simulink model "DTNS"  (R2022a)
settings: Solver=FixedStepDiscrete  StartTime=0.0  StopTime=0.4  FixedStep=0.04  RelTol=1e-3
PreLoadFcn:
  | listing = dir;
  | if (contains([listing.name], 'MAP')) &&  (contains([listing.name], 'DTNS.slx'))
  |     addpath('./AGR', './TRN', './TCAF', './MAP');
  |     addpath('./MAP/MAP_DB');
  | else
  |     warning('[DTNS.slx]는 DTNS 프로젝트 최상단 경로에 위치해야 합니다.');
  | end
  | 
  | load('BusStructureTRN.mat');
  | load('BusStructureLOSR.mat');
  | load('BusStructureHR.mat');
  | load('BusStructureCR.mat');
InitFcn:
  | listing = dir;
  | if (contains([listing.name], 'MAP')) &&  (contains([listing.name], 'DTNS.slx'))
  |     addpath('./AGR', './TRN', './TCAF', './MAP');
  |     addpath('./MAP/MAP_DB');
  | else
  |     warning('[DTNS.slx]는 DTNS 프로젝트 최상단 경로에 위치해야 합니다.');
  | end
  | 
  | load('BusStructureTRN.mat');
  | load('BusStructureLOSR.mat');
  | load('BusStructureHR.mat');
  | load('BusStructureCR.mat');
settings Model: Creator=ASCL  LastModifiedBy=ASCL
settings SolverCC: PositivePriorityOrder=on
settings DataIOCC: SaveOutput=off  SignalLogging=off  DSMLogging=off  SaveTime=off  ReturnWorkspaceOutputs=off
settings OptimizationCC: BlockReduction=off  DefaultParameterBehavior=Inlined  UseDivisionForNetSlopeComputation=on  GainParamInheritBuiltInType=on  UseFloatMulNetSlope=on  ExpressionFolding=off  PassReuseOutputArgsAs=Individual arguments  ZeroExternalMemoryAtStartup=off  ZeroInternalMemoryAtStartup=off  EfficientFloat2IntCast=on  LifeSpan=Inf  OptimizeBlockOrder=speed  DifferentSizesBufferReuse=on  EfficientTunableParamExpr=on
settings DebuggingCC: SignalInfNanChecking=warning  ReadBeforeWriteMsg=EnableAllAsError  WriteAfterWriteMsg=EnableAllAsError  WriteAfterReadMsg=EnableAllAsError  IntegerOverflowMsg=error  ParameterTunabilityLossMsg=error  UniqueDataStoreMsg=error  AssertControl=DisableAll  NonBusSignalsTreatedAsBus=error  SFInvalidInputDataAccessInChartInitDiag=error  SFTransitionOutsideNaturalParentDiag=error  SFUnreachableExecutionPathDiag=error  SFUndirectedBroadcastEventsDiag=error  IntegerSaturationMsg=error
settings HardwareCC: ProdBitPerPointer=32  ProdBitPerSizeT=32  ProdBitPerPtrDiffT=32  ProdLargestAtomicInteger=Long  ProdLargestAtomicFloat=Double  ProdEndianess=BigEndian  ProdWordSize=32  ProdLongLongMode=on  ProdHWDeviceType=Freescale->MPC83xx
settings ModelReferenceCC: ModelReferenceNumInstancesAllowed=Single  PropagateSignalLabelsOutOfModel=off
settings SFSimCC: SimCustomHeaderCode="#include \"MAP.h\""  SimUserSources=MAP.c  SimUserLibraries=WS2_32.LIB  CompileTimeRecursionLimit=0  EnableRuntimeRecursion=off  MATLABDynamicMemAlloc=off
settings RTWCC: SystemTargetFile=ert.tlc  TemplateMakefile=ert_default_tmf  GenerateReport=on  RTWUseSimCustomCode=on  CustomHeaderCode="#include \"MAP.h\""  CustomSource=MAP.c  CustomLibrary=WS2_32.LIB  BuildConfiguration=Faster Runs  IncludeHyperlinkInReport=on  LaunchReport=on  GenerateTraceInfo=on  GenerateTraceReport=on  GenerateTraceReportSl=on  GenerateTraceReportSf=on  GenerateTraceReportEml=on  GenerateCodeMetricsReport=on
settings CodeAppCC: ForceParamTrailComments=on  IgnoreCustomStorageClasses=off  OperatorAnnotations=on  SimulinkDataObjDesc=on  SFDataObjDesc=on  MATLABFcnDesc=on  InsertBlockDesc=on  StateflowObjectComments=on  MATLABSourceComments=on  EnableCustomComments=on  InlinedPrmAccess=Macros  ReqsInCode=on
settings ERTTargetCC: TargetLangStandard=C99 (ISO)  UtilityFuncGeneration=Shared location  GenerateSampleERTMain=on  CombineSignalStateStructs=on  SuppressErrorStatus=on  SupportNonFinite=off  SupportVariableSizeSignals=on  ParenthesesLevel=Standards  CastingMode=Standards  GenerateSharedConstants=off  InlinedParameterPlacement=NonHierarchical  ERTCustomFileTemplate=example_file_process.tlc  RateTransitionBlockCode=Function  PreserveIfCondition=on  ConvertIfToSwitch=off  EnableSignedLeftShifts=off  EnableSignedRightShifts=off

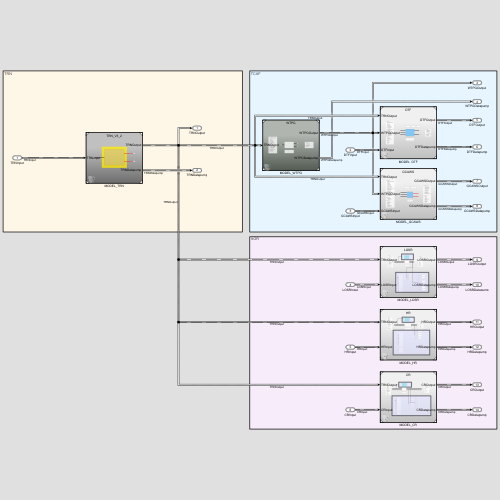
[thumbnail: Simulink's stored preview of the top-level diagram]
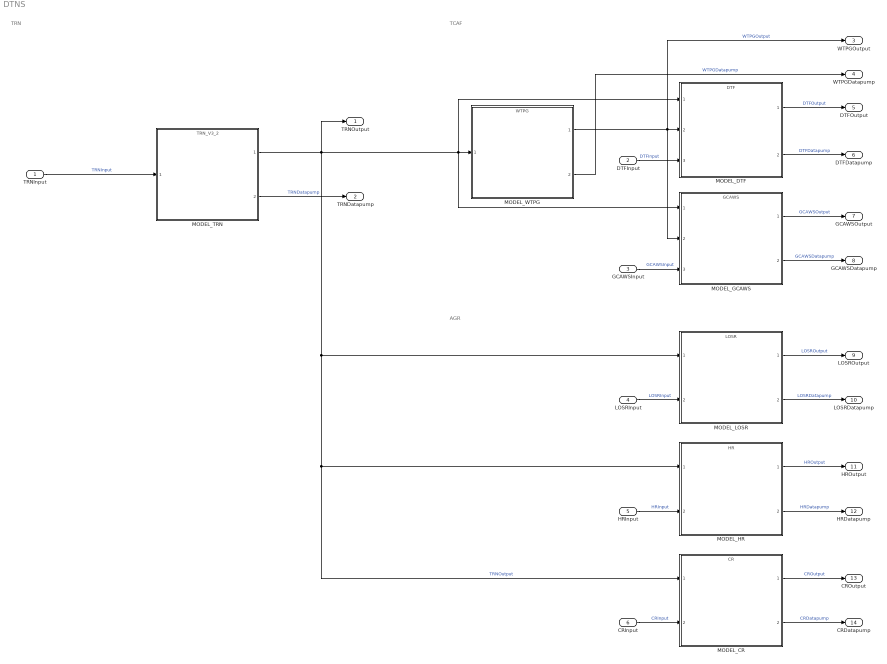
== system DTNS ==
  note: TRN
  note: AGR
  note: TCAF
  TRNInput : Inport  OutDataTypeStr=Bus: TRNInput  SampleTime=0.04  Interpolate=off  BusOutputAsStruct=on
  DTFInput : Inport  Port=2  OutDataTypeStr=Bus: DTFInput  SampleTime=0.04  Interpolate=off  BusOutputAsStruct=on
  GCAWSInput : Inport  Port=3  OutDataTypeStr=Bus: GCAWSInput  SampleTime=0.04  Interpolate=off  BusOutputAsStruct=on
  LOSRInput : Inport  Port=4  OutDataTypeStr=Bus: LOSRInput  SampleTime=0.04  Interpolate=off  BusOutputAsStruct=on
  HRInput : Inport  Port=5  OutDataTypeStr=Bus: HRInput  SampleTime=0.04  Interpolate=off  BusOutputAsStruct=on
  CRInput : Inport  Port=6  OutDataTypeStr=Bus: CRInput  SampleTime=0.04  Interpolate=off  BusOutputAsStruct=on
  MODEL_CR : ModelReference  ModelNameDialog=CR.slx  SimulationMode=Normal  ModelReferenceVersion=1.261
  MODEL_DTF : ModelReference  ModelNameDialog=DTF.slx  SimulationMode=Normal  ModelReferenceVersion=1.441
  MODEL_GCAWS : ModelReference  ModelNameDialog=GCAWS.slx  SimulationMode=Normal  ModelReferenceVersion=1.799
  MODEL_HR : ModelReference  ModelNameDialog=HR.slx  SimulationMode=Normal  ModelReferenceVersion=1.387
  MODEL_LOSR : ModelReference  ModelNameDialog=LOSR.slx  SimulationMode=Normal  ModelReferenceVersion=1.367
  MODEL_TRN : ModelReference  ModelNameDialog=TRN_V3_2.slx  SimulationMode=Normal  ModelReferenceVersion=2.356
  MODEL_WTPG : ModelReference  ModelNameDialog=WTPG.slx  SimulationMode=Normal  CachedPortDiscreteRates=[0.04]  ModelReferenceVersion=1.390
  TRNOutput : Outport  OutDataTypeStr=Bus: TRNOutput  SampleTime=0.04  BusOutputAsStruct=on
  TRNDatapump : Outport  Port=2  OutDataTypeStr=Bus: TRNDatapump  SampleTime=0.04
  WTPGOutput : Outport  Port=3  OutDataTypeStr=Bus: WTPGOutput  SampleTime=0.04
  WTPGDatapump : Outport  Port=4  OutDataTypeStr=Bus: WTPGDatapump  SampleTime=0.04
  DTFOutput : Outport  Port=5  OutDataTypeStr=Bus: DTFOutput  SampleTime=0.04
  DTFDatapump : Outport  Port=6  OutDataTypeStr=Bus: DTFDatapump  SampleTime=0.04
  GCAWSOutput : Outport  Port=7  OutDataTypeStr=Bus: GCAWSOutput  SampleTime=0.04
  GCAWSDatapump : Outport  Port=8  OutDataTypeStr=Bus: GCAWSDatapump  SampleTime=0.04
  LOSROutput : Outport  Port=9  OutDataTypeStr=Bus: LOSROutput  SampleTime=0.04  BusOutputAsStruct=on
  LOSRDatapump : Outport  Port=10  OutDataTypeStr=Bus: LOSRDatapump  SampleTime=0.04  BusOutputAsStruct=on
  HROutput : Outport  Port=11  OutDataTypeStr=Bus: HROutput  SampleTime=0.04  BusOutputAsStruct=on
  HRDatapump : Outport  Port=12  OutDataTypeStr=Bus: HRDatapump  SampleTime=0.04  BusOutputAsStruct=on
  CROutput : Outport  Port=13  OutDataTypeStr=Bus: CROutput  SampleTime=0.04  BusOutputAsStruct=on
  CRDatapump : Outport  Port=14  OutDataTypeStr=Bus: CRDatapump  SampleTime=0.04  BusOutputAsStruct=on
  wires:
  MODEL_WTPG/2 -> WTPGDatapump/1  "WTPGDatapump"
  TRNInput/1 -> MODEL_TRN/1  "TRNInput"
  MODEL_DTF/1 -> DTFOutput/1  "DTFOutput"
  MODEL_GCAWS/1 -> GCAWSOutput/1  "GCAWSOutput"
  MODEL_TRN/2 -> TRNDatapump/1  "TRNDatapump"
  MODEL_DTF/2 -> DTFDatapump/1  "DTFDatapump"
  MODEL_GCAWS/2 -> GCAWSDatapump/1  "GCAWSDatapump"
  MODEL_WTPG/1 -> MODEL_GCAWS/2, MODEL_DTF/2, WTPGOutput/1  "WTPGOutput"
  MODEL_TRN/1 -> MODEL_CR/1, MODEL_HR/1, MODEL_LOSR/1, TRNOutput/1, MODEL_GCAWS/1, MODEL_WTPG/1, MODEL_DTF/1  "TRNOutput"
  DTFInput/1 -> MODEL_DTF/3  "DTFInput"
  GCAWSInput/1 -> MODEL_GCAWS/3  "GCAWSInput"
  LOSRInput/1 -> MODEL_LOSR/2  "LOSRInput"
  HRInput/1 -> MODEL_HR/2  "HRInput"
  CRInput/1 -> MODEL_CR/2  "CRInput"
  MODEL_LOSR/1 -> LOSROutput/1  "LOSROutput"
  MODEL_LOSR/2 -> LOSRDatapump/1  "LOSRDatapump"
  MODEL_HR/1 -> HROutput/1  "HROutput"
  MODEL_HR/2 -> HRDatapump/1  "HRDatapump"
  MODEL_CR/1 -> CROutput/1  "CROutput"
  MODEL_CR/2 -> CRDatapump/1  "CRDatapump"
